simulink model "generadorSenalCuadradaFourier"  (R2015a)
settings: Solver=ode45  StartTime=0.0  StopTime=2*pi  MaxStep=0.0025  MinStep=0.0025  RelTol=0.0025  AbsTol=0.0025
settings Model: Creator=Javi  LastModifiedBy=Javi
settings SolverCC: InitialStep=0

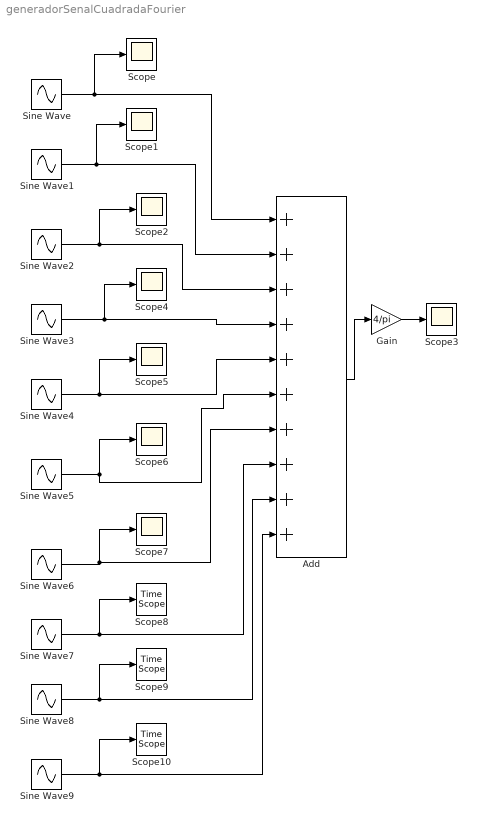
== system generadorSenalCuadradaFourier ==
  Add : Sum  Inputs=++++++++++
  Gain : Gain  Gain=4/pi
  Scope{,1..7} (8 alike) : Scope
      Scope settings: TimeRange=1  YMin=0  YMax=0.3
      Scope1 settings: TimeRange=1  YMin=0.332081  YMax=0.364605
      Scope2 settings: TimeRange=1  YMin=0  YMax=0.3  SaveName=ScopeData2
      Scope3 settings: TimeRange=1  YMin=0  YMax=0.3  SaveName=ScopeData3
      Scope4 settings: TimeRange=1  YMin=0  YMax=0.3  SaveName=ScopeData4
      Scope5 settings: TimeRange=1  YMin=0  YMax=0.3  SaveName=ScopeData5
      Scope6 settings: TimeRange=1  YMin=0  YMax=0.3  SaveName=ScopeData6
      Scope7 settings: TimeRange=1  YMin=0  YMax=0.3  SaveName=ScopeData7
  Scope10 : TimeScope
  Scope8 : TimeScope
  Scope9 : TimeScope
  Sine Wave : Sin  SampleTime=0
  Sine Wave1 : Sin  Amplitude=1/3  Frequency=3  SampleTime=0
  Sine Wave2 : Sin  Amplitude=1/5  Frequency=5  SampleTime=0
  Sine Wave3 : Sin  Amplitude=1/7  Frequency=7  SampleTime=0
  Sine Wave4 : Sin  Amplitude=1/9  Frequency=9  SampleTime=0
  Sine Wave5 : Sin  Amplitude=1/11  Frequency=11  SampleTime=0
  Sine Wave6 : Sin  Amplitude=1/13  Frequency=13  SampleTime=0
  Sine Wave7 : Sin  Amplitude=1/15  Frequency=15  SampleTime=0
  Sine Wave8 : Sin  Amplitude=1/17  Frequency=17  SampleTime=0
  Sine Wave9 : Sin  Amplitude=1/19  Frequency=19  SampleTime=0
  wires:
  Sine Wave/1 -> Add/1, Scope/1
  Sine Wave1/1 -> Add/2, Scope1/1
  Sine Wave2/1 -> Add/3, Scope2/1
  Gain/1 -> Scope3/1
  Sine Wave3/1 -> Add/4, Scope4/1
  Sine Wave4/1 -> Add/5, Scope5/1
  Sine Wave5/1 -> Scope6/1, Add/6
  Sine Wave6/1 -> Add/7, Scope7/1
  Add/1 -> Gain/1
  Sine Wave7/1 -> Add/8, Scope8/1
  Sine Wave8/1 -> Add/9, Scope9/1
  Sine Wave9/1 -> Add/10, Scope10/1
